simulink model "acados_test"  (R2018b)
settings: Solver=FixedStepDiscrete  StartTime=0.0  StopTime=400  FixedStep=0.5  RelTol=1e-3
PostLoadFcn:
  | , if any(exist('dsrtsu_mdlpostloadfcn', 'file') == [2, 3, 6]), try dsrtsu_mdlpostloadfcn('Execute', bdroot); catch fprintf('Error in PostLoadFcn (dsrtsu_mdlpostloadfcn) for model "%s":\n %s\n', bdroot, lasterr); end, end,
settings Model: DSRTSU_INTERNAL_RTI_VER=520  DSRTSU_INTERNAL_RTI_TYPE=rti1401  RTICANMMDATA=struct('GeneralSetupData',struct('modelroot','D:\dSpace_Acados_Test','generalsettings',struct('filesettings',struct('destfolder',struct('Name','RTICANMM_FILES','Check',1),'buildfolder',struct('Name','.','Check',1),'AbsDestfolder',struct('Name','D:\dSpace_Acados_Test\RTICANMM_FILES'),'AbsBuildfolder',struct('Name','D:\dSpace_Acados_Test'))),'options',struct('addpaths',1,'rmpaths',1,'addtrcexclusion',logical(1),'cannavigator',struct('checkmonitoring',0),'show_usrtrc',0,'use_usrtrc',0),'advanced',struct('options',ones(1,100)),'MPSetup',{{}},'RTI',struct('Type','RTI1401','Ver','7.10','Date','02-May-2018'),'modelname','acados_test','block','acados_test'))  Creator=oj  LastModifiedBy=fleqscar
settings SolverCC: AlgebraicLoopSolver=LineSearch
settings DataIOCC: ReturnWorkspaceOutputs=on
settings OptimizationCC: BlockReduction=off  OptimizeBlockIOStorage=off  BufferReuse=off  LocalBlockOutputs=off  InitFltsAndDblsToZero=on  EfficientMapNaN2IntZero=off  BufferReusableBoundary=off
settings HardwareCC: ProdBitPerPointer=32  ProdBitPerSizeT=32  ProdBitPerPtrDiffT=32  ProdLargestAtomicInteger=Integer  ProdEndianess=BigEndian  ProdWordSize=32  ProdHWDeviceType=Custom Processor->Custom  TargetIntDivRoundTo=Zero  TargetEndianess=BigEndian  TargetHWDeviceType=Custom Processor->Custom
settings SFSimCC: MATLABDynamicMemAlloc=off
settings RTWCC: Description=dSPACE DS1401 Hardware Platform  SystemTargetFile=rti1401.tlc  MakeCommand=make_rti  TemplateMakefile=rti1401.tmf  BuildConfiguration=Debug
settings CodeAppCC: ForceParamTrailComments=on  MATLABSourceComments=on
settings STFCustomTargetCC: ParMdlRefBuildCompliant=on  SystemTargetFile=rti1401.tlc
settings GRTTargetCC: TargetLangStandard=C89/C90 (ANSI)  CompOptLevelCompliant=off  ConcurrentExecutionCompliant=off  CombineOutputUpdateFcns=off  MatFileLogging=off  CPPClassGenCompliant=off  UseToolchainInfoCompliant=off

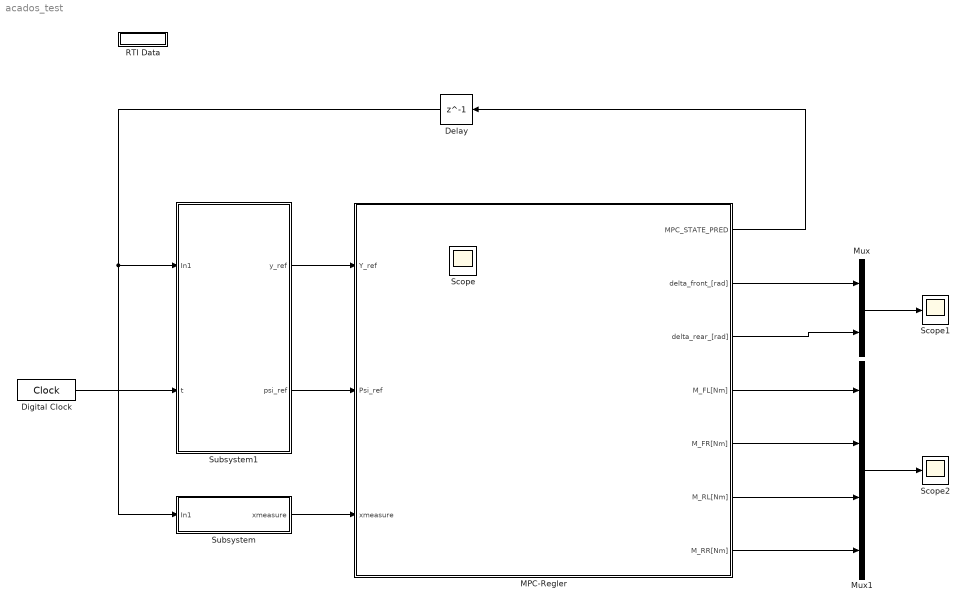
== system acados_test ==
  Delay : Delay  DelayLength=1
  Digital Clock : DigitalClock  SampleTime=-1
  MPC-Regler : Subsystem
  Mux : Mux  Inputs=2
  Mux1 : Mux
  RTI Data : Subsystem  Tag=struct('RTIDataServer',struct('RTIDataServerVs','2','RTIModelDescription','struct(''main'',''acados_test'',''sub'',''acados_test'',''isMp'',0)'))  LoadFcn="if exist('rtidc'), try,  rtidc('DataHostBlockClbLoad', gcbh); catch, disp(['Warning: ''LoadFcn'' for RTI Data block failed: ' lasterr]); end, end,"  mask(RTI_DATA_HOST){}
      mask help:
      | RTI Data Block.
      | This block is used by RTI to store internal model-dependent data.
      | Please keep this block on the root level of the model. Deleting this block will result in data loss.
      |
      | NEVER DELETE OR COPY THIS BLOCK!
      settings: CopyFcn="if exist('rtidc'), try,  rtidc('DataHostBlockClbCopy', gcbh); catch, disp(['Warning: ''CopyFcn'' for RTI Data block failed: ' lasterr]); end, end,"  DeleteFcn="if exist('rtidc'), try,  rtidc('DataHostBlockClbDelete', gcbh); catch, disp(['Warning: ''DeleteFcn'' for RTI Data block failed: ' lasterr]); end, end,"  ModelCloseFcn="if exist('rtidc'), try,  rtidc('DataHostBlockClbModelClose', gcbh); catch, disp(['Warning: ''ModelCloseFcn'' for RTI Data block failed: ' lasterr]); end, end,"  PreSaveFcn="if exist('rtidc'), try,  rtidc('DataHostBlockClbPreSave', gcbh); catch, disp(['Warning: ''PreSaveFcn'' for RTI Data block failed: ' lasterr]); end, end,"  PostSaveFcn="if exist('rtidc'), try,  rtidc('DataHostBlockClbPostSave', gcbh); catch, disp(['Warning: ''PostSaveFcn'' for RTI Data block failed: ' lasterr]); end, end,"  NameChangeFcn="if exist('rtidc'), try,  rtidc('DataHostBlockClbNameChange', gcbh); catch, disp(['Warning: ''NameChangeFcn'' for RTI Data block failed: ' lasterr]); end, end,"
      mask Help:
      | RTI Data Block.
      | This block is used by RTI to store internal model-dependent data.
      | Please keep this block on the root level of the model. Deleting this block will result in data loss.
      | 
      | NEVER DELETE OR COPY THIS BLOCK!
      mask Display: text(0.5, 0.5, 'RTI Data', 'HorizontalAlignment', 'center');
  Scope1 : Scope
  Scope2 : Scope
  Subsystem : Subsystem
  Subsystem1 : Subsystem  InitFcn=x_pred = 0:0.1:4.9;
  Scope : Scope
  wires:
  Mux/1 -> Scope1/1
  Delay/1 -> Subsystem/1(In1), Subsystem1/1(In1)
  Mux1/1 -> Scope2/1
  MPC-Regler/3(" delta_rear_[rad]") -> Mux/2
  MPC-Regler/2(" delta_front_[rad]") -> Mux/1
  MPC-Regler/1(MPC_STATE_PRED) -> Delay/1
  MPC-Regler/4(M_FL[Nm]) -> Mux1/1
  MPC-Regler/5(M_FR[Nm]) -> Mux1/2
  MPC-Regler/6(M_RL[Nm]) -> Mux1/3
  MPC-Regler/7(M_RR[Nm]) -> Mux1/4
  Subsystem1/1(y_ref) -> MPC-Regler/1(Y_ref)
  Subsystem1/2(psi_ref) -> MPC-Regler/2(Psi_ref)
  Subsystem/1(xmeasure) -> MPC-Regler/3(xmeasure)
  Digital Clock/1 -> Subsystem1/2(t)

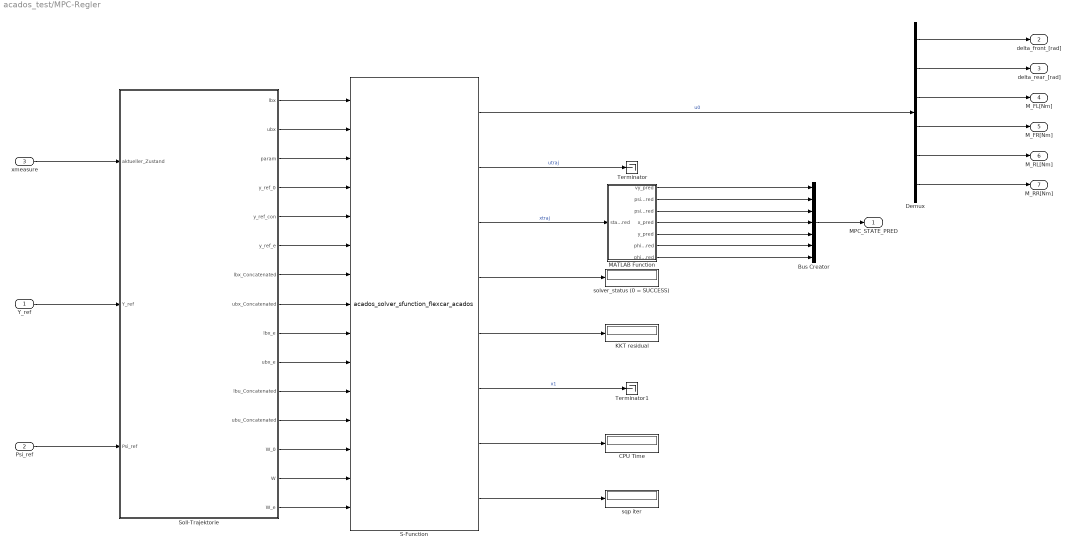
== system acados_test/MPC-Regler ==
  Y_ref : Inport
  Psi_ref : Inport  Port=2
  xmeasure : Inport  Port=3
  Bus Creator : BusCreator  Inputs=7
  CPU Time : Display
  Demux : Demux  Outputs=6
  KKT residual : Display
  MATLAB Function : MATLAB Function  TreatAsAtomicUnit=on
  S-Function : S-Function  FunctionName=acados_solver_sfunction_flexcar_acados  SFunctionDeploymentMode=off  EnableBusSupport=off
  Soll-Trajektorie : Subsystem
  Terminator : Terminator
  Terminator1 : Terminator
  solver_status (0 = SUCCESS) : Display
  sqp iter : Display
  MPC_STATE_PRED : Outport  VectorParamsAs1DForOutWhenUnconnected=off
  " delta_front_[rad]" : Outport  Port=2  VectorParamsAs1DForOutWhenUnconnected=off
  " delta_rear_[rad]" : Outport  Port=3  VectorParamsAs1DForOutWhenUnconnected=off
  M_FL[Nm] : Outport  Port=4  VectorParamsAs1DForOutWhenUnconnected=off
  M_FR[Nm] : Outport  Port=5  VectorParamsAs1DForOutWhenUnconnected=off
  M_RL[Nm] : Outport  Port=6  VectorParamsAs1DForOutWhenUnconnected=off
  M_RR[Nm] : Outport  Port=7  VectorParamsAs1DForOutWhenUnconnected=off
  wires:
  Soll-Trajektorie/10(ubx_e) -> S-Function/10
  Soll-Trajektorie/9(lbx_e) -> S-Function/9
  Soll-Trajektorie/4(y_ref_0) -> S-Function/4
  Soll-Trajektorie/15(W_e) -> S-Function/15
  Soll-Trajektorie/6(y_ref_e) -> S-Function/6
  Soll-Trajektorie/2(ubx) -> S-Function/2
  Soll-Trajektorie/7(lbx_Concatenated) -> S-Function/7
  Soll-Trajektorie/12(ubu_Concatenated) -> S-Function/12
  Soll-Trajektorie/3(param) -> S-Function/3
  Soll-Trajektorie/8(ubx_Concatenated) -> S-Function/8
  Soll-Trajektorie/13(W_0) -> S-Function/13
  Soll-Trajektorie/1(lbx) -> S-Function/1
  Soll-Trajektorie/11(lbu_Concatenated) -> S-Function/11
  Soll-Trajektorie/5(y_ref_con) -> S-Function/5
  Soll-Trajektorie/14(W) -> S-Function/14
  xmeasure/1 -> Soll-Trajektorie/1(aktueller_Zustand)
  Y_ref/1 -> Soll-Trajektorie/2(Y_ref)
  Psi_ref/1 -> Soll-Trajektorie/3(Psi_ref)
  S-Function/7 -> CPU Time/1
  Demux/2 -> " delta_rear_[rad]"/1
  Demux/1 -> " delta_front_[rad]"/1
  Demux/4 -> M_FR[Nm]/1
  S-Function/2 -> Terminator/1  "utraj"
  MATLAB Function/7(phi_pred) -> Bus Creator/7
  Bus Creator/1 -> MPC_STATE_PRED/1
  S-Function/4 -> solver_status (0 = SUCCESS)/1
  MATLAB Function/1(vy_pred) -> Bus Creator/1
  S-Function/8 -> sqp iter/1
  S-Function/1 -> Demux/1  "u0"
  S-Function/6 -> Terminator1/1  "x1"
  MATLAB Function/4(x_pred) -> Bus Creator/4
  MATLAB Function/6(phidot_pred) -> Bus Creator/6
  MATLAB Function/2(psidot_pred) -> Bus Creator/2
  S-Function/3 -> MATLAB Function/1(state_pred)  "xtraj"
  Demux/3 -> M_FL[Nm]/1
  MATLAB Function/3(psi_pred) -> Bus Creator/3
  Demux/6 -> M_RR[Nm]/1
  Demux/5 -> M_RL[Nm]/1
  S-Function/5 -> KKT residual/1
  MATLAB Function/5(y_pred) -> Bus Creator/5

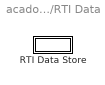
== system acados_test/RTI Data ==
  RTI Data Store : Subsystem  mask(RTI_DATA_STORE){}
      mask help:
      | RTI Data Store Block. This block is used by RTI to store internal model dependent data. Deleting this block will result in data loss.
      |
      | NEVER DELETE, COPY, OR MODIFY THIS BLOCK!
      mask Help:
      | RTI Data Store Block. This block is used by RTI to store internal model dependent data. Deleting this block will result in data loss.
      | 
      | NEVER DELETE, COPY, OR MODIFY THIS BLOCK!
      mask Display: text(0.5, 0.5, ' ', 'HorizontalAlignment', 'center');

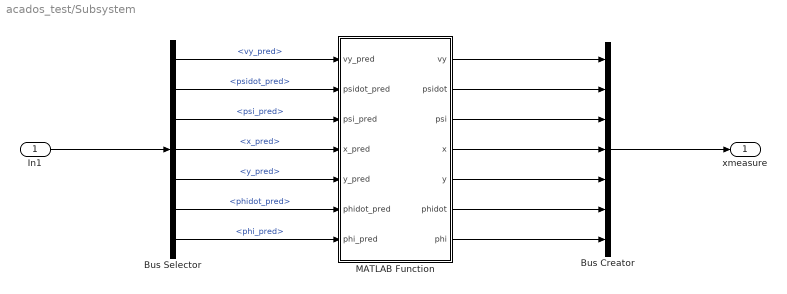
== system acados_test/Subsystem ==
  In1 : Inport
  Bus Creator : BusCreator  Inputs=7
  Bus Selector : BusSelector  OutputSignals=vy_pred,psidot_pred,psi_pred,x_pred,y_pred,phidot_pred,phi_pred
  MATLAB Function : MATLAB Function  TreatAsAtomicUnit=on
  xmeasure : Outport  VectorParamsAs1DForOutWhenUnconnected=off
  wires:
  In1/1 -> Bus Selector/1
  Bus Selector/1 -> MATLAB Function/1(vy_pred)  "<vy_pred>"
  Bus Selector/2 -> MATLAB Function/2(psidot_pred)  "<psidot_pred>"
  Bus Selector/3 -> MATLAB Function/3(psi_pred)  "<psi_pred>"
  Bus Selector/4 -> MATLAB Function/4(x_pred)  "<x_pred>"
  Bus Selector/5 -> MATLAB Function/5(y_pred)  "<y_pred>"
  Bus Selector/6 -> MATLAB Function/6(phidot_pred)  "<phidot_pred>"
  Bus Selector/7 -> MATLAB Function/7(phi_pred)  "<phi_pred>"
  MATLAB Function/1(vy) -> Bus Creator/1
  MATLAB Function/2(psidot) -> Bus Creator/2
  MATLAB Function/3(psi) -> Bus Creator/3
  MATLAB Function/4(x) -> Bus Creator/4
  MATLAB Function/5(y) -> Bus Creator/5
  MATLAB Function/6(phidot) -> Bus Creator/6
  MATLAB Function/7(phi) -> Bus Creator/7
  Bus Creator/1 -> xmeasure/1

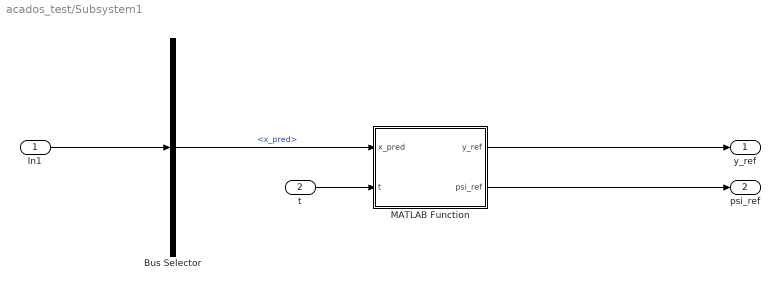
== system acados_test/Subsystem1 ==
  In1 : Inport
  t : Inport  Port=2
  Bus Selector : BusSelector  OutputSignals=x_pred
  MATLAB Function : MATLAB Function  TreatAsAtomicUnit=on
  y_ref : Outport  VectorParamsAs1DForOutWhenUnconnected=off
  psi_ref : Outport  Port=2  VectorParamsAs1DForOutWhenUnconnected=off
  wires:
  In1/1 -> Bus Selector/1
  Bus Selector/1 -> MATLAB Function/1(x_pred)  "<x_pred>"
  MATLAB Function/1(y_ref) -> y_ref/1
  MATLAB Function/2(psi_ref) -> psi_ref/1
  t/1 -> MATLAB Function/2(t)

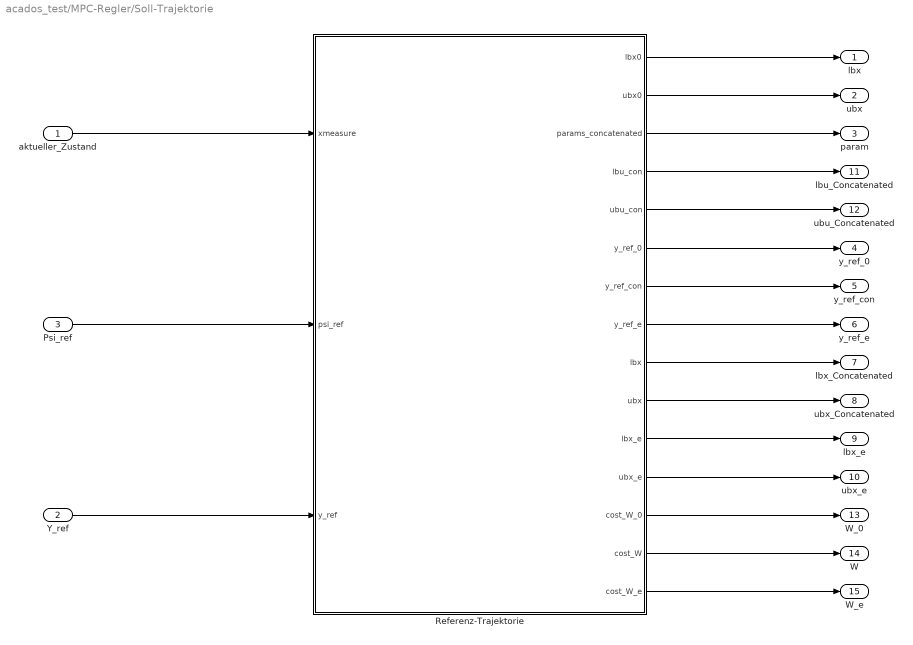
== system acados_test/MPC-Regler/Soll-Trajektorie ==
  aktueller_Zustand : Inport
  Y_ref : Inport  Port=2
  Psi_ref : Inport  Port=3
  Referenz-Trajektorie : MATLAB Function  TreatAsAtomicUnit=on
  lbx : Outport  VectorParamsAs1DForOutWhenUnconnected=off
  ubx : Outport  Port=2  VectorParamsAs1DForOutWhenUnconnected=off
  param : Outport  Port=3  VectorParamsAs1DForOutWhenUnconnected=off
  y_ref_0 : Outport  Port=4  VectorParamsAs1DForOutWhenUnconnected=off
  y_ref_con : Outport  Port=5  VectorParamsAs1DForOutWhenUnconnected=off
  y_ref_e : Outport  Port=6  VectorParamsAs1DForOutWhenUnconnected=off
  lbx_Concatenated : Outport  Port=7  VectorParamsAs1DForOutWhenUnconnected=off
  ubx_Concatenated : Outport  Port=8  VectorParamsAs1DForOutWhenUnconnected=off
  lbx_e : Outport  Port=9  VectorParamsAs1DForOutWhenUnconnected=off
  ubx_e : Outport  Port=10  VectorParamsAs1DForOutWhenUnconnected=off
  lbu_Concatenated : Outport  Port=11  VectorParamsAs1DForOutWhenUnconnected=off
  ubu_Concatenated : Outport  Port=12  VectorParamsAs1DForOutWhenUnconnected=off
  W_0 : Outport  Port=13  VectorParamsAs1DForOutWhenUnconnected=off
  W : Outport  Port=14  VectorParamsAs1DForOutWhenUnconnected=off
  W_e : Outport  Port=15  VectorParamsAs1DForOutWhenUnconnected=off
  wires:
  aktueller_Zustand/1 -> Referenz-Trajektorie/1(xmeasure)
  Referenz-Trajektorie/3(params_concatenated) -> param/1
  Psi_ref/1 -> Referenz-Trajektorie/2(psi_ref)
  Y_ref/1 -> Referenz-Trajektorie/3(y_ref)
  Referenz-Trajektorie/5(ubu_con) -> ubu_Concatenated/1
  Referenz-Trajektorie/4(lbu_con) -> lbu_Concatenated/1
  Referenz-Trajektorie/6(y_ref_0) -> y_ref_0/1
  Referenz-Trajektorie/7(y_ref_con) -> y_ref_con/1
  Referenz-Trajektorie/8(y_ref_e) -> y_ref_e/1
  Referenz-Trajektorie/15(cost_W_e) -> W_e/1
  Referenz-Trajektorie/14(cost_W) -> W/1
  Referenz-Trajektorie/13(cost_W_0) -> W_0/1
  Referenz-Trajektorie/9(lbx) -> lbx_Concatenated/1
  Referenz-Trajektorie/10(ubx) -> ubx_Concatenated/1
  Referenz-Trajektorie/11(lbx_e) -> lbx_e/1
  Referenz-Trajektorie/12(ubx_e) -> ubx_e/1
  Referenz-Trajektorie/1(lbx0) -> lbx/1
  Referenz-Trajektorie/2(ubx0) -> ubx/1

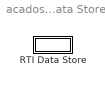
== system acados_test/RTI Data/RTI Data Store ==
  RTI Data Store : Subsystem  mask(RTI_DATA_STORE){}
      mask help:
      | RTI Data Store Block. This block is used by RTI to store internal model dependent data. Deleting this block will result in data loss.
      |
      | NEVER DELETE, COPY, OR MODIFY THIS BLOCK!
      mask Help:
      | RTI Data Store Block. This block is used by RTI to store internal model dependent data. Deleting this block will result in data loss.
      | 
      | NEVER DELETE, COPY, OR MODIFY THIS BLOCK!
      mask Display: text(0.5, 0.5, ' ', 'HorizontalAlignment', 'center');

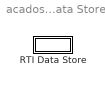
== system acados_test/RTI Data/RTI Data Store/RTI Data Store ==
  RTI Data Store : Subsystem  mask(RTI_DATA_STORE){}
      mask help:
      | RTI Data Store Block. This block is used by RTI to store internal model dependent data. Deleting this block will result in data loss.
      |
      | NEVER DELETE, COPY, OR MODIFY THIS BLOCK!
      mask Help:
      | RTI Data Store Block. This block is used by RTI to store internal model dependent data. Deleting this block will result in data loss.
      | 
      | NEVER DELETE, COPY, OR MODIFY THIS BLOCK!
      mask Display: text(0.5, 0.5, ' ', 'HorizontalAlignment', 'center');

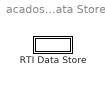
== system acados_test/RTI Data/RTI Data Store/RTI Data Store/RTI Data Store ==
  RTI Data Store : Subsystem  mask(RTI_DATA_STORE){}
      mask help:
      | RTI Data Store Block. This block is used by RTI to store internal model dependent data. Deleting this block will result in data loss.
      |
      | NEVER DELETE, COPY, OR MODIFY THIS BLOCK!
      mask Help:
      | RTI Data Store Block. This block is used by RTI to store internal model dependent data. Deleting this block will result in data loss.
      | 
      | NEVER DELETE, COPY, OR MODIFY THIS BLOCK!
      mask Display: text(0.5, 0.5, ' ', 'HorizontalAlignment', 'center');

== system acados_test/RTI Data/RTI Data Store/RTI Data Store/RTI Data Store/RTI Data Store ==

== matlab function acados_test/MPC-Regler/MATLAB Function ==
  data: state_pred input; vy_pred output; psidot_pred output; psi_pred output; x_pred output; y_pred output; phidot_pred output; phi_pred output
function [vy_pred, psidot_pred, psi_pred, x_pred, y_pred, phidot_pred, phi_pred] = fcn(state_pred)

N = 50;
st_pred = reshape(state_pred, 7, N+1);

vy_pred = st_pred(1, 1:N);
psidot_pred = st_pred(2, 1:N);
psi_pred = st_pred(3, 1:N);
x_pred = st_pred(4, 1:N);
y_pred = st_pred(5, 1:N);
phidot_pred = st_pred(6, 1:N);
phi_pred = st_pred(7, 1:N);

end

== matlab function acados_test/MPC-Regler/Soll-Trajektorie/Referenz-Trajektorie ==
  data: lbx0 output size=[1, 7]; ubx0 output size=[1, 7]; xmeasure input size=[1, 7]; psi_ref input size=[1, 50]; y_ref input size=[1, 50]; params_concatenated output size=[1, 153]; lbu_con output; ubu_con output; y_ref_0 output; y_ref_con output; y_ref_e output; lbx output size=[1, 98]; ubx output size=[1, 98]; lbx_e output size=[1, 2]; ubx_e output size=[1, 2]; cost_W_0 output size=[1, 196]; cost_W output size=[1, 196]; cost_W_e output size=[1, 49]
function [lbx0, ubx0, params_concatenated, lbu_con, ubu_con, y_ref_0, y_ref_con, y_ref_e, ...
          lbx, ubx, lbx_e, ubx_e, cost_W_0, cost_W, cost_W_e]  = fcn(xmeasure, psi_ref, y_ref)

lbx0 = xmeasure; 
ubx0 = xmeasure; 
      
lbu = [-deg2rad(23),-deg2rad(23), -50, -50, -50, -50]';
param = [1.5349e+05, 1.56618e+05, 0.3775, 100, 0.315, 1, 1e-4, 1e-2, 2, 2, 3e-7, 3e-7, 3e-7, 3e-7, 10];
nx = 7; 
nu = 6;
n_M = 1; 
nz = 0;
N = 50;

Fx_ref = param(4);
rdyn = param(5);

vx = param(15);

Q_11 = param(6); 
Q_22 = param(7); 
Q_33 = param(8); 
R_11 = param(9); 
R_22 = param(10); 
R_33 = param(11); 
R_44 = param(12); 
R_55 = param(13); 
R_66 = param(14); 

param0 = [Fx_ref; rdyn; vx];
params_concatenated = repmat(param0, N+1, 1)';

lbu_con = repmat(lbu, N, 1);
ubu_con = -lbu_con;


%% Ref for Optimization Variable Y = [X; U]
y_ref_0 = zeros(nx+nu+n_M, 1);
y_ref_0(3) = psi_ref(1);
y_ref_0(5) = y_ref(1);
y_ref_0(end) = Fx_ref;

y_ref_mat = zeros(nx+nu+n_M, N-1);
y_ref_mat(3, :) = psi_ref(2:end);
y_ref_mat(5, :) = y_ref(2:end);
y_ref_mat(end, :) = Fx_ref * ones(1, N-1)';
y_ref_con = reshape(y_ref_mat, (nx+nu+n_M)*(N-1), 1);

y_ref_e = zeros(nx, 1);
y_ref_e(3) = psi_ref(end);
y_ref_e(5) = y_ref(end);

Y_ref_lb = zeros(2, N-1);
Y_ref_ub = zeros(2, N-1);
Y_ref_lb(1, :) = y_ref_mat(3, :) - deg2rad(30); % -10deg 
Y_ref_lb(2, :) = y_ref_mat(5, :) - 1;         % -0.1m
Y_ref_ub(1, :) = y_ref_mat(3, :) + deg2rad(30); % +10deg 
Y_ref_ub(2, :) = y_ref_mat(5, :) + 1;         % +0.1m

% Reshape in column-major form (thats what reshape() does!)
lbx = reshape(Y_ref_lb, 1, 2*(N-1));
ubx = reshape(Y_ref_ub, 1, 2*(N-1));
lbx_e = [y_ref_e(3), y_ref_e(5)];
ubx_e = [y_ref_e(3), y_ref_e(5)];

%% WEIGHTING MATRICES
% W_x = diag([0; 0; p(3); 0; p(4); 0; 0]);
% W_u = diag(p(6:11));
% W_Mx = p(5);

COST_W_0 = zeros(nx+nu+n_M, nx+nu+n_M);
COST_W_e = zeros(nx, nx);

COST_W_0(3, 3) = Q_11;
COST_W_0(5, 5) = Q_22;
COST_W_0(8:13, 8:13) = diag([R_11, R_22, R_33, R_44, R_55, R_66]);
COST_W_0(14, 14) = Q_33;

COST_W_e = 10*COST_W_0(1:nx, 1:nx);

% Reshape in column-major form (thats what reshape() does!)
cost_W_0 = reshape(COST_W_0, 1, (nx+nu+n_M)*(nx+nu+n_M));
cost_W = cost_W_0;
cost_W_e = reshape(COST_W_e, 1, nx*nx);

== matlab function acados_test/Subsystem/MATLAB Function ==
  data: vy output; psidot output; psi output; x output; vy_pred input size=[1, 50]; y output; psidot_pred input size=[1, 50]; psi_pred input size=[1, 50]; x_pred input size=[1, 50]; y_pred input size=[1, 50]; phidot_pred input size=[1, 50]; phi_pred input size=[1, 50]; phidot output; phi output
function [vy, psidot, psi, x, y, phidot, phi] = fcn(vy_pred, psidot_pred, psi_pred, x_pred, y_pred, phidot_pred, phi_pred)

vy = vy_pred(2);
psidot = psidot_pred(2);
psi = psi_pred(2);
x = x_pred(2);
y = y_pred(2);
phidot = phidot_pred(2);
phi = phi_pred(2);



end

== matlab function acados_test/Subsystem1/MATLAB Function ==
  data: x_pred input; y_ref output size=[1, 50]; psi_ref output size=[1, 50]; t input
function [y_ref, psi_ref] = fcn(x_pred, t)

if t < 0.025
    x_pred = 0:0.1:4.9;
end
Y_ref = @(x) sin(0.1*x);
Psi_ref = @(x) 0.1*cos(0.1*x);

y_ref = Y_ref(x_pred);
psi_ref = Psi_ref(x_pred);

end
